simulink model "simlag"  (Simulink 7.9)
settings: Solver=ode45  StartTime=0.0  StopTime=10.0  RelTol=1e-3
values from neighbouring files (symbols this model uses):
  Ax = 0.25    [Constantes_simulink.m]
  Ay = 0.25    [Constantes_simulink.m]
  Az = 0.25    [Constantes_simulink.m]
  b = 1.14E-7    (= 1.14e-07)    [Constantes_simulink.m]
  g = 9.81    [Constantes_simulink.m]
  Ixx = 0.004856    [Constantes_simulink.m]
  Iyy = 0.004856    [Constantes_simulink.m]
  Izz = 0.008801    [Constantes_simulink.m]
  k = 0.00000298    (= 2.98e-06)    [Constantes_simulink.m]
  l = 0.225    [Constantes_simulink.m]
  m = 0.468    [Constantes_simulink.m]
settings Model: Creator=gabriel  LastModifiedBy=gabriel
settings DebuggingCC: SolverPrmCheckMsg=none

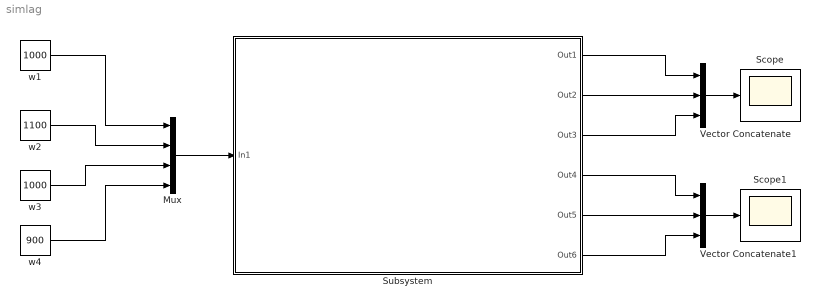
== system simlag ==
  Mux : Mux
  Scope : Scope
      settings: TickLabels=on  ShowLegends=on
  Scope1 : Scope
  Subsystem : Subsystem
      mask Display: image(imread('Quad.jpeg'))
  Vector Concatenate : Concatenate  NumInputs=3
  Vector Concatenate1 : Concatenate  NumInputs=3
  w1 : Constant  Value=1000
  w2 : Constant  Value=1100
  w3 : Constant  Value=1000
  w4 : Constant  Value=900
  wires:
  w1/1 -> Mux/1
  w2/1 -> Mux/2
  w3/1 -> Mux/3
  w4/1 -> Mux/4
  Mux/1 -> Subsystem/1(In1)
  Subsystem/1(Out1) -> Vector Concatenate/1
  Subsystem/2(Out2) -> Vector Concatenate/2
  Subsystem/3(Out3) -> Vector Concatenate/3
  Vector Concatenate/1 -> Scope/1
  Subsystem/4(Out4) -> Vector Concatenate1/1
  Subsystem/5(Out5) -> Vector Concatenate1/2
  Subsystem/6(Out6) -> Vector Concatenate1/3
  Vector Concatenate1/1 -> Scope1/1

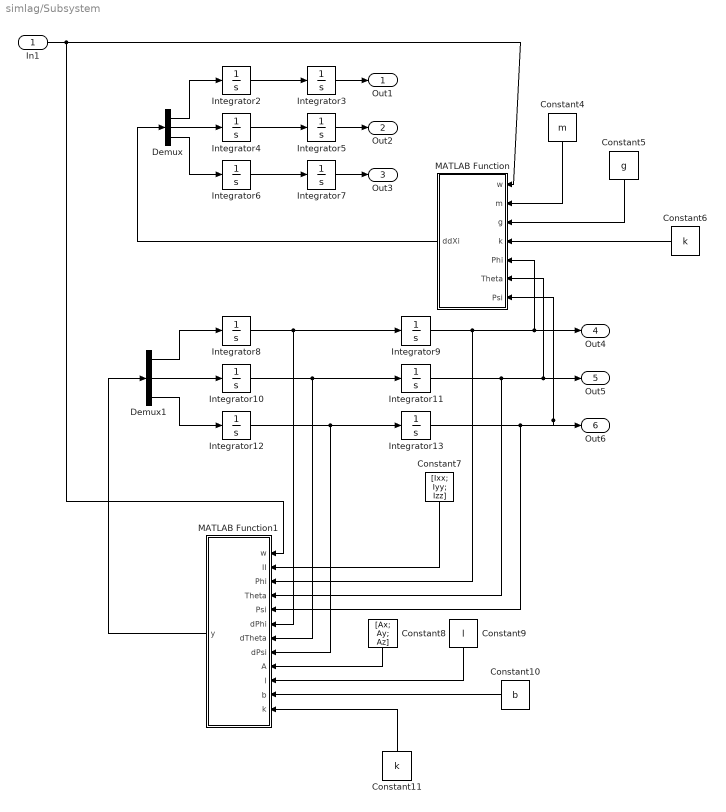
== system simlag/Subsystem ==
  In1 : Inport
  Constant10 : Constant  Value=b
  Constant11 : Constant  Value=k
  Constant4 : Constant  Value=m
  Constant5 : Constant  Value=g
  Constant6 : Constant  Value=k
  Constant7 : Constant  Value=[Ixx; Iyy; Izz]
  Constant8 : Constant  Value=[Ax; Ay; Az]
  Constant9 : Constant  Value=l
  Demux : Demux  Outputs=3
  Demux1 : Demux  Outputs=3
  Integrator{2..13} (12 alike) : Integrator
  MATLAB Function : MATLAB Function  TreatAsAtomicUnit=on
  MATLAB Function1 : MATLAB Function  TreatAsAtomicUnit=on
  Out1 : Outport
  Out2 : Outport  Port=2
  Out3 : Outport  Port=3
  Out4 : Outport  Port=4
  Out5 : Outport  Port=5
  Out6 : Outport  Port=6
  wires:
  Integrator2/1 -> Integrator3/1
  Integrator4/1 -> Integrator5/1
  Integrator6/1 -> Integrator7/1
  Integrator8/1 -> Integrator9/1, MATLAB Function1/6(dPhi)
  Integrator10/1 -> Integrator11/1, MATLAB Function1/7(dTheta)
  Integrator12/1 -> Integrator13/1, MATLAB Function1/8(dPsi)
  In1/1 -> MATLAB Function1/1(w), MATLAB Function/1(w)
  Integrator9/1 -> MATLAB Function1/3(Phi), MATLAB Function/5(Phi), Out4/1
  Integrator11/1 -> MATLAB Function1/4(Theta), MATLAB Function/6(Theta), Out5/1
  Integrator13/1 -> MATLAB Function1/5(Psi), MATLAB Function/7(Psi), Out6/1
  Constant4/1 -> MATLAB Function/2(m)
  Constant5/1 -> MATLAB Function/3(g)
  Constant6/1 -> MATLAB Function/4(k)
  MATLAB Function/1(ddXi) -> Demux/1
  Demux/1 -> Integrator2/1
  Demux/2 -> Integrator4/1
  Demux/3 -> Integrator6/1
  Constant7/1 -> MATLAB Function1/2(II)
  Demux1/1 -> Integrator8/1
  Demux1/2 -> Integrator10/1
  Demux1/3 -> Integrator12/1
  MATLAB Function1/1(y) -> Demux1/1
  Constant8/1 -> MATLAB Function1/9(A)
  Constant9/1 -> MATLAB Function1/10(l)
  Constant10/1 -> MATLAB Function1/11(b)
  Constant11/1 -> MATLAB Function1/12(k)
  Integrator3/1 -> Out1/1
  Integrator5/1 -> Out2/1
  Integrator7/1 -> Out3/1

== matlab function Subsystem/MATLAB Function1 ==
  data: w input double; y output double; II input double; Phi input double; Theta input double; Psi input double; dPhi input double; dTheta input double; dPsi input double; A input double; l input double; b input double; k input double
function y = fcn(w,II,Phi,Theta,Psi,dPhi,dTheta,dPsi,A,l,b,k)
%#codegen

Ixx=II(1);
Iyy=II(2);
Izz=II(3);

TauB=[[l*k*(w(4)^2-w(2)^2)];
      [l*k*(w(3)^2-w(1)^2)];
      [b*(w(1)^2+w(3)^2-w(2)^2-w(4)^2)]];

Weta=[[1 0 -sin(Theta)];
      [0 cos(Phi) cos(Theta)*sin(Phi)];
      [0 -sin(Phi) cos(Theta)*cos(Phi)]];
 
J=transpose(Weta)*[[Ixx 0 0];[0 Iyy 0];[0 0 Izz]]*Weta;  

% CdEta=[((Izz*sin(2*Phi)*cos(Theta)^2)/2 - (Iyy*sin(2*Phi)*cos(Theta)^2)/2)*dPsi^2 + (Izz*cos(2*Phi)*cos(Theta) - Iyy*cos(2*Phi)*cos(Theta) - Ixx*cos(Theta))*dPsi*dTheta + ((Iyy*sin(2*Phi))/2 - (Izz*sin(2*Phi))/2)*dTheta^2;
%        dPsi^2*(Izz*cos(Phi)^2*cos(Theta)*sin(Theta) - Ixx*cos(Theta)*sin(Theta) + Iyy*cos(Theta)*sin(Phi)^2*sin(Theta)) - ddTheta*(Iyy*cos(Phi)^2 + Izz*sin(Phi)^2) - ddPsi*(Iyy*cos(Phi)*cos(Theta)*sin(Phi) - Izz*cos(Phi)*cos(Theta)*sin(Phi)) + Iyy*ddTheta*cos(Phi)^2 + Izz*ddTheta*sin(Phi)^2 - dPhi*dTheta*(2*Iyy*cos(Phi)*sin(Phi) - 2*Izz*cos(Phi)*sin(Phi)) + dPhi*dPsi*(Ixx*cos(Theta) + Iyy*cos(Phi)^2*cos(Theta) - Izz*cos(Phi)^2*cos(Theta) - Iyy*cos(Theta)*sin(Phi)^2 + Izz*cos(Theta)*sin(Phi)^2) + Iyy*ddPsi*cos(Phi)*cos(Theta)*sin(Phi) - Izz*ddPsi*cos(Phi)*cos(Theta)*sin(Phi);
%        Ixx*ddPsi*sin(Theta)^2 - ddPsi*(Izz*cos(Phi)^2*cos(Theta)^2 + Iyy*cos(Theta)^2*sin(Phi)^2 + Ixx*sin(Theta)^2) - ddTheta*(Iyy*cos(Phi)*cos(Theta)*sin(Phi) - Izz*cos(Phi)*cos(Theta)*sin(Phi)) - dTheta^2*(Iyy*cos(Phi)*sin(Phi)*sin(Theta) - Izz*cos(Phi)*sin(Phi)*sin(Theta)) - dPsi*dTheta*(2*Izz*cos(Phi)^2*cos(Theta)*sin(Theta) - 2*Ixx*cos(Theta)*sin(Theta) + 2*Iyy*cos(Theta)*sin(Phi)^2*sin(Theta)) - dPhi*dTheta*(Ixx*cos(Theta) - Iyy*cos(Phi)^2*cos(Theta) + Izz*cos(Phi)^2*cos(Theta) + Iyy*cos(Theta)*sin(Phi)^2 - Izz*cos(Theta)*sin(Phi)^2) + dPhi*dPsi*(2*Iyy*cos(Phi)*cos(Theta)^2*sin(Phi) - 2*Izz*cos(Phi)*cos(Theta)^2*sin(Phi)) + Izz*ddPsi*cos(Phi)^2*cos(Theta)^2 + Iyy*ddPsi*cos(Theta)^2*sin(Phi)^2 + Iyy*ddTheta*cos(Phi)*cos(Theta)*sin(Phi) - Izz*ddTheta*cos(Phi)*cos(Theta)*sin(Phi)]
 
% CdEta=[(Iyy*dTheta^2*sin(2*Phi))/2 - (Izz*dTheta^2*sin(2*Phi))/2 - Ixx*dPsi*dTheta*cos(Theta) - (Iyy*dPsi^2*sin(2*Phi)*cos(Theta)^2)/2 + (Izz*dPsi^2*sin(2*Phi)*cos(Theta)^2)/2 - Iyy*dPsi*dTheta*cos(2*Phi)*cos(Theta) + Izz*dPsi*dTheta*cos(2*Phi)*cos(Theta);
%         dPhi*(Ixx*dPsi*cos(Theta) - 2*Iyy*dTheta*cos(Phi)*sin(Phi) + 2*Izz*dTheta*cos(Phi)*sin(Phi) + Iyy*dPsi*cos(Phi)^2*cos(Theta) - Izz*dPsi*cos(Phi)^2*cos(Theta) - Iyy*dPsi*cos(Theta)*sin(Phi)^2 + Izz*dPsi*cos(Theta)*sin(Phi)^2) - Ixx*dPsi^2*cos(Theta)*sin(Theta) + Iyy*dPsi^2*cos(Theta)*sin(Phi)^2*sin(Theta) + Izz*dPsi^2*cos(Phi)^2*cos(Theta)*sin(Theta);
%         -dPhi*(Ixx*dTheta*cos(Theta) - Iyy*dTheta*cos(Phi)^2*cos(Theta) + Izz*dTheta*cos(Phi)^2*cos(Theta) + Iyy*dTheta*cos(Theta)*sin(Phi)^2 - Izz*dTheta*cos(Theta)*sin(Phi)^2 - 2*Iyy*dPsi*cos(Phi)*cos(Theta)^2*sin(Phi) + 2*Izz*dPsi*cos(Phi)*cos(Theta)^2*sin(Phi))  - Iyy*dTheta^2*cos(Phi)*sin(Phi)*sin(Theta) + Izz*dTheta^2*cos(Phi)*sin(Phi)*sin(Theta) + 2*Ixx*dPsi*dTheta*cos(Theta)*sin(Theta) - 2*Izz*dPsi*dTheta*cos(Phi)^2*cos(Theta)*sin(Theta) - 2*Iyy*dPsi*dTheta*cos(Theta)*sin(Phi)^2*sin(Theta)];    


  CdEta=[(Iyy*dTheta^2*sin(2*Phi))/2 - (Izz*dTheta^2*sin(2*Phi))/2 - Ixx*dPsi*dTheta*cos(Theta) - (Iyy*dPsi^2*sin(2*Phi)*cos(Theta)^2)/2 + (Izz*dPsi^2*sin(2*Phi)*cos(Theta)^2)/2 - Iyy*dPsi*dTheta*cos(2*Phi)*cos(Theta) + Izz*dPsi*dTheta*cos(2*Phi)*cos(Theta);
          dPhi*(Ixx*dPsi*cos(Theta) - 2*Iyy*dTheta*cos(Phi)*sin(Phi) + 2*Izz*dTheta*cos(Phi)*sin(Phi) + Iyy*dPsi*cos(Phi)^2*cos(Theta) - Izz*dPsi*cos(Phi)^2*cos(Theta) - Iyy*dPsi*cos(Theta)*sin(Phi)^2 + Izz*dPsi*cos(Theta)*sin(Phi)^2)  - Ixx*dPsi^2*cos(Theta)*sin(Theta) + Iyy*dPsi^2*cos(Theta)*sin(Phi)^2*sin(Theta)  + Izz*dPsi^2*cos(Phi)^2*cos(Theta)*sin(Theta);
          -dPhi*(Ixx*dTheta*cos(Theta) - Iyy*dTheta*cos(Phi)^2*cos(Theta) + Izz*dTheta*cos(Phi)^2*cos(Theta) + Iyy*dTheta*cos(Theta)*sin(Phi)^2 - Izz*dTheta*cos(Theta)*sin(Phi)^2 - 2*Iyy*dPsi*cos(Phi)*cos(Theta)^2*sin(Phi) + 2*Izz*dPsi*cos(Phi)*cos(Theta)^2*sin(Phi))  - Iyy*dTheta^2*cos(Phi)*sin(Phi)*sin(Theta) + Izz*dTheta^2*cos(Phi)*sin(Phi)*sin(Theta) + 2*Ixx*dPsi*dTheta*cos(Theta)*sin(Theta) - 2*Izz*dPsi*dTheta*cos(Phi)^2*cos(Theta)*sin(Theta) - 2*Iyy*dPsi*dTheta*cos(Theta)*sin(Phi)^2*sin(Theta)];
y = inv(J)*(TauB-CdEta);

== matlab function Subsystem/MATLAB Function ==
  data: w input double; m input double; g input double; k input double; Phi input double; Theta input double; Psi input double; ddXi output double
function ddXi = fcn(w,m,g,k,Phi,Theta,Psi)
%#codegen

R=[[cos(Psi)*cos(Theta) cos(Psi)*sin(Theta)*sin(Phi)-sin(Psi)*cos(Phi) cos(Psi)*sin(Theta)*cos(Phi)+sin(Psi)*sin(Phi)];
   [sin(Psi)*cos(Theta) sin(Psi)*sin(Theta)*sin(Phi)+cos(Psi)*cos(Phi) sin(Psi)*sin(Theta)*cos(Phi)-cos(Psi)*sin(Phi)];
   [-sin(Theta) cos(Theta)*sin(Phi) cos(Theta)*cos(Phi)]];

T=[0; 0; k*(w(1)^2+w(2)^2+w(3)^2+w(4)^2)/m];

ddXi = R*T+[0; 0; -g];
